simulink model "simexa30"  (Simulink 4.00)
settings: Solver=ode45  SolverMode=SingleTasking  StartTime=0.0  StopTime=10  RelTol=1e-3  AbsTol=1e-6
settings Model: LastModifiedBy=saadat  LimitDataPoints=off  RTWTemplateMakefile=grt_vc.tmf  ExtModeTrigMode=oneshot  ExtModeArmWhenConnect=off

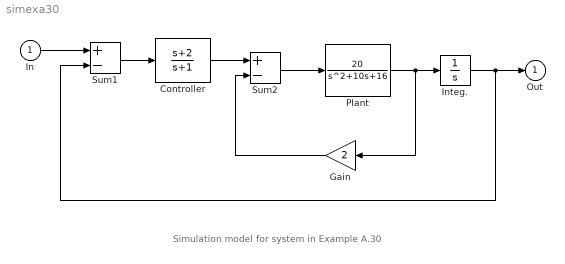
== system simexa30 ==
  note: Simulation model for system in Example A.30
  In : Inport  Port=1  LatchInput=off
  Controller : TransferFcn  Numerator=[1 2]  Denominator=[1 1]  AbsoluteTolerance=auto  Realization=auto
  Gain : Gain  Orientation=left  Gain=2  Multiplication=Element-wise(K.*u)  SaturateOnIntegerOverflow=on
  Integ. : Integrator  ExternalReset=none  InitialConditionSource=internal  InitialCondition=0  LimitOutput=off  UpperSaturationLimit=inf  LowerSaturationLimit=-inf  ShowSaturationPort=off  ShowStatePort=off  AbsoluteTolerance=auto
  Plant : TransferFcn  Numerator=[20]  Denominator=[1 10 16]  AbsoluteTolerance=auto  Realization=auto
  Sum1 : Sum  Inputs=+-  SaturateOnIntegerOverflow=on
  Sum2 : Sum  Inputs=+-  SaturateOnIntegerOverflow=on
  Out : Outport  Port=1
  wires:
  Integ./1 -> Sum1/2, Out/1
  In/1 -> Sum1/1
  Controller/1 -> Sum2/1
  Sum1/1 -> Controller/1
  Plant/1 -> Gain/1, Integ./1
  Gain/1 -> Sum2/2
  Sum2/1 -> Plant/1
